simulink model "estimate_eci_vecs_test"  (R2016b)
settings: Solver=VariableStepAuto  StartTime=0.0  StopTime=1080  RelTol=1e-3
undefined symbols (not defined in the file): Earth, fsw_params, WGS84
libraries: tle2eci_coarse_lib x2, aerolibtransform2 x1, gps x1, GPS_processing_lib x1, MSP_FSW_lib x1, mag_vec_lib x1, sgp4_lib_fsw x1, eci_2_TLE_lib x1
settings Model: Creator=Taylor  LastModifiedBy=Taylor

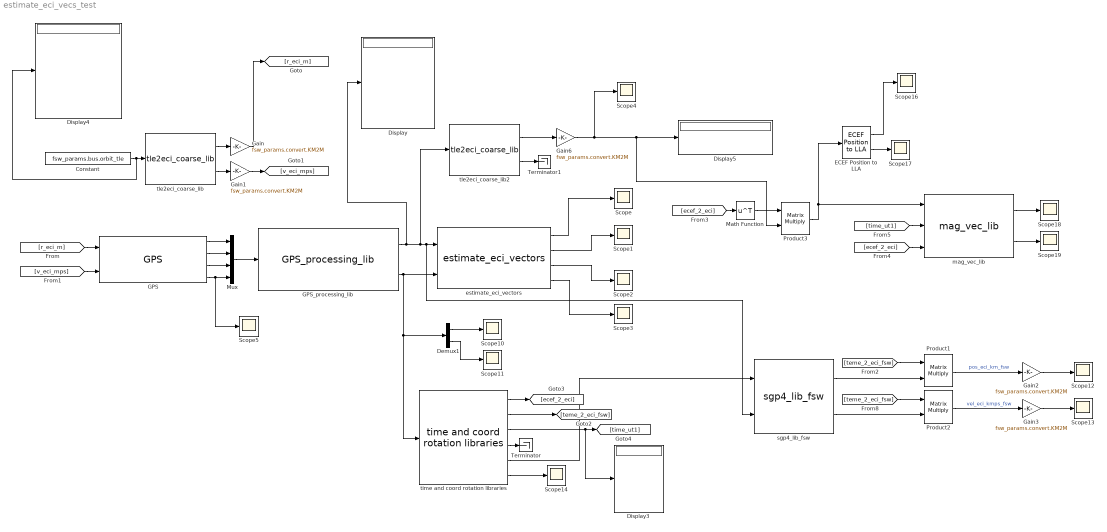
== system estimate_eci_vecs_test ==
  Constant : Constant  Value=fsw_params.bus.orbit_tle
  Demux1 : Demux  Outputs=2
  Display{,3..5} (4 alike) : Display
  ECEF Position to LLA : aerolibtransform2/ECEF Position to LLA  units=Metric (MKS)  ptype=Earth (WGS84)  F=1/298.257223563  R=6378137
  GPS : gps/GPS
  GPS_processing_lib : GPS_processing_lib/GPS_processing_lib
  Gain{,1..3,6} (5 alike) : Gain  Gain=fsw_params.convert.KM2M
  Math Function : Math  Operator=transpose  SaturateOnIntegerOverflow=on
  Mux : Mux  Inputs=[3 3 2 1]
  Product1 : Product  Multiplication=Matrix(*)
  Product2 : Product  Multiplication=Matrix(*)
  Product3 : Product  Multiplication=Matrix(*)
  Scope{,1..5,10..14,16..19} (15 alike) : Scope
  Terminator : Terminator
  Terminator1 : Terminator
  estimate_eci_vectors : MSP_FSW_lib/MSP_FSW/estimate_eci_vectors
  mag_vec_lib : mag_vec_lib/mag_vec_lib
  sgp4_lib_fsw : sgp4_lib_fsw/sgp4_lib_fsw
  time and coord rotation libraries : eci_2_TLE_lib/eci_2_TLE_lib/time and coord rotation libraries
  tle2eci_coarse_lib : tle2eci_coarse_lib/tle2eci_coarse_lib
  tle2eci_coarse_lib2 : tle2eci_coarse_lib/tle2eci_coarse_lib
  wires:
  Mux/1 -> GPS_processing_lib/1
  estimate_eci_vectors/1 -> Scope/1
  estimate_eci_vectors/2 -> Scope1/1
  estimate_eci_vectors/3 -> Scope2/1
  estimate_eci_vectors/4 -> Scope3/1
  GPS/1 -> Mux/1
  GPS/2 -> Mux/2
  GPS/3 -> Mux/3
  GPS/4 -> Scope5/1, Mux/4
  tle2eci_coarse_lib/1 -> Gain/1
  tle2eci_coarse_lib/2 -> Gain1/1
  Constant/1 -> Display4/1, tle2eci_coarse_lib/1
  Gain/1 -> [r_eci_m]
  Gain1/1 -> [v_eci_mps]
  [r_eci_m] -> GPS/1
  [v_eci_mps] -> GPS/2
  GPS_processing_lib/2 -> estimate_eci_vectors/2, Demux1/1, time and coord rotation libraries/1
  Demux1/1 -> Scope10/1
  Demux1/2 -> Scope11/1
  time and coord rotation libraries/1 -> [ecef_2_eci]
  time and coord rotation libraries/4 -> Terminator/1
  time and coord rotation libraries/3 -> Display3/1, [time_ut1]
  time and coord rotation libraries/6 -> Scope14/1
  [teme_2_eci_fsw] -> Product1/1
  [teme_2_eci_fsw] -> Product2/1
  time and coord rotation libraries/5 -> sgp4_lib_fsw/1
  Product2/1 -> Gain3/1  "vel_eci_kmps_fsw"
  sgp4_lib_fsw/2 -> Product2/2
  sgp4_lib_fsw/1 -> Product1/2
  Product1/1 -> Gain2/1  "pos_eci_km_fsw"
  time and coord rotation libraries/2 -> [teme_2_eci_fsw]
  Gain3/1 -> Scope13/1
  Gain2/1 -> Scope12/1
  GPS_processing_lib/1 -> sgp4_lib_fsw/2, estimate_eci_vectors/1, tle2eci_coarse_lib2/1, Display/1
  Math Function/1 -> Product3/1
  [ecef_2_eci] -> Math Function/1
  Product3/1 -> mag_vec_lib/1, ECEF Position to LLA/1
  ECEF Position to LLA/2 -> Scope17/1
  ECEF Position to LLA/1 -> Scope16/1
  [ecef_2_eci] -> mag_vec_lib/3
  [time_ut1] -> mag_vec_lib/2
  mag_vec_lib/1 -> Scope18/1
  mag_vec_lib/2 -> Scope19/1
  tle2eci_coarse_lib2/1 -> Gain6/1
  Gain6/1 -> Scope4/1, Product3/2, Display5/1
  tle2eci_coarse_lib2/2 -> Terminator1/1
